simulink model "wlan80211BeaconRx"  (R2018a)
settings: Solver=FixedStepDiscrete  StartTime=0.0  StopTime=Inf  RelTol=1e-3
InitFcn:
  | wlan80211BeaconRxModelParams
  | load('wlan80211BusTypes.mat')
StartFcn:
  | wlan80211BeaconRxModelParams
  | load('wlan80211BusTypes.mat')
model workspace: external: MAT-File (data not in the file)
values from neighbouring files (symbols this model uses):
  p80211 = commwlan80211BeaconRxInit(agcStepSize, agcMaxGain,      corrThreshold, sampsPerChip)    [wlan80211BeaconRxModelParams.m]
libraries: commwlan80211BeaconLib x3, commsync2 x2, commdigbbndpm3 x1, commsequence2 x1, commrfcorlib x1, dspsigops x1, commfilt2 x1
CloseFcn:
  | hFig = findall(0, 'Type', 'figure', 'Name', '802.11 Beacon Frame');
  | if ishghandle(hFig)
  | close(hFig);
  | end
  | clear hFig
  | if (exist('ans')==1) && (iscell(ans) && (numel(ans) == 0))
  | clear ans
  | end
Description:
  | IEEE 802.11 WLAN Beacon Frame Receiver for Captured Data
  | 
  | This example shows how to process a captured beacon frame and display the
  | frame information.
settings Model: Creator=The MathWorks, Inc.  LastModifiedBy=minh
settings DataIOCC: LimitDataPoints=on  SaveFormat=Array  SaveOutput=off  SignalLogging=off  DSMLogging=off  SaveTime=off
settings OptimizationCC: DefaultParameterBehavior=Inlined  InlineInvariantSignals=on  ExpressionDepthLimit=2147483647  EfficientFloat2IntCast=on  LifeSpan=inf
settings DebuggingCC: UnderspecifiedInitializationDetection=Classic  MergeDetectMultiDrivingBlocksExec=none  SolverPrmCheckMsg=warning  UniqueDataStoreMsg=error  AllowSymbolicDim=off  StateNameClashWarn=warning  SFUnexpectedBacktrackingDiag=warning  SFNoUnconditionalDefaultTransitionDiag=warning  SFExecutionAtInitializationDiag=none
settings HardwareCC: ProdBitPerPointer=32  ProdBitPerSizeT=32  ProdBitPerPtrDiffT=32  ProdLargestAtomicFloat=None  ProdIntDivRoundTo=Undefined  ProdEndianess=Unspecified  ProdWordSize=32  ProdHWDeviceType=32-bit Generic
settings ModelReferenceCC: PropagateSignalLabelsOutOfModel=off
settings CodeAppCC: StateflowObjectComments=on
settings GRTTargetCC: TargetLangStandard=C89/C90 (ANSI)  GeneratePreprocessorConditionals=Disable all  CombineOutputUpdateFcns=off  GRTInterface=on
settings ConfigComp: CovMetricSettings=dw  CovHtmlReporting=on  CovSaveCumulativeToWorkspaceVar=on  CovSaveSingleToWorkspaceVar=on  CovShowResultsExplorer=off  CovExternalEMLEnable=off  CovSFcnEnable=off

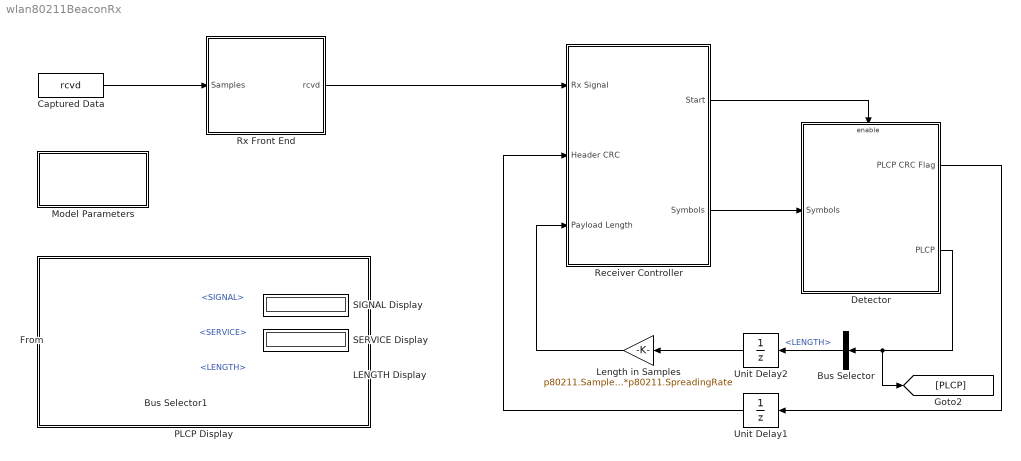
== system wlan80211BeaconRx ==
  Bus Selector : BusSelector  OutputSignals=LENGTH
  Bus Selector1 : BusSelector  OutputSignals=SIGNAL,SERVICE,LENGTH
  Captured Data : FromWorkspace  VariableName=rcvd  SampleTime=p80211.SamplesPerChannelFrame / (p80211.ChipRate*p80211.SamplesPerChip)  Interpolate=off  OutputAfterFinalValue=Cyclic repetition
  Detector : Subsystem
      settings: CloseFcn=clear BeaconFrameBodyType rcvd
  LENGTH Display : Display
  Length in Samples : Gain  Gain=p80211.SamplesPerChip*p80211.SpreadingRate  OutDataTypeStr=uint32  SaturateOnIntegerOverflow=on  ParamDataTypeStr=Inherit: Same as input
  Model Parameters : Subsystem  mask(Model Parameters){rcvdSignal=Channel 5, agcStepSize=6, agcMaxGain=60, corrThreshold=500, sampsPerChip=2}
      mask prompts: rcvdSignal "Received signal:"; agcStepSize "AGC loop gain:"; agcMaxGain "Maximum AGC power gain in dB:"; corrThreshold "Synchronization threshold:"; sampsPerChip "Samples per chip:"
      mask help:
      | Choose 802.11 receiver parameters.
      |
      | You can select from four different saved received signals that contain 802.11 packets captured using a radio.
      |
      | You can set the AGC parameters and samples per chip used in the receiver. You can also set the synchronization threshold value to determine the correlation threshold used to declare the presence of an 802.11 packet.
      mask init:
      | commwlan80211BeaconRxModelParams('init');
      mask Help: helpview(commdhelp);
      mask TypeOptions rcvdSignal: Channel 5 | Channel 9
      mask TypeOptions sampsPerChip: 4 | 2
      mask Display: disp('Model\nParameters')
  PLCP Display : Subsystem
      mask Display: disp('')
  Receiver Controller : Subsystem
  Rx Front End : Subsystem
  SERVICE Display : Display
      settings: Format=hex (Stored Integer)
  SIGNAL Display : Display
      settings: Format=hex (Stored Integer)
  Unit Delay1 : UnitDelay  InitialCondition=1  SampleTime=-1
  Unit Delay2 : UnitDelay  InitialCondition=1  SampleTime=-1
  wires:
  Length in Samples/1 -> Receiver Controller/3(Payload Length)
  Detector/1(PLCP CRC Flag) -> Unit Delay1/1
  Unit Delay1/1 -> Receiver Controller/2(Header CRC)
  Bus Selector/1 -> Unit Delay2/1  "<LENGTH>"
  Receiver Controller/1(Start) -> Detector/Enable
  Rx Front End/1(rcvd) -> Receiver Controller/1(Rx Signal)
  Unit Delay2/1 -> Length in Samples/1
  Detector/2(PLCP) -> [PLCP], Bus Selector/1
  [PLCP] -> Bus Selector1/1
  Bus Selector1/3 -> LENGTH Display/1  "<LENGTH>"
  Bus Selector1/1 -> SIGNAL Display/1  "<SIGNAL>"
  Bus Selector1/2 -> SERVICE Display/1  "<SERVICE>"
  Receiver Controller/2(Symbols) -> Detector/1(Symbols)
  Captured Data/1 -> Rx Front End/1(Samples)

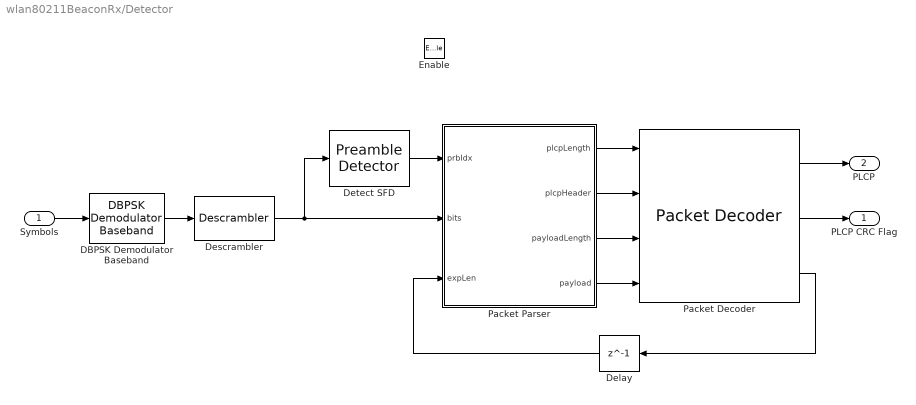
== system wlan80211BeaconRx/Detector ==
  Symbols : Inport
  Enable : EnablePort  StatesWhenEnabling=reset  PropagateVarSize=During execution
  DBPSK Demodulator Baseband : commdigbbndpm3/DBPSK Demodulator Baseband  Ph=0  outDtype=Smallest unsigned integer
      settings: SourceProductName=Communications System Toolbox  SourceProductBaseCode=CM
  Delay : Delay  DelayLength=1  InitialCondition=0  InputProcessing=Columns as channels (frame based)
  Descrambler : commsequence2/Descrambler  M=2  poly=p80211.ScramblerPolynomial  iniStaSource=Dialog Parameter  ini_sta=[0 0 0 0 0 0 0]  resetViaPort=off
      settings: SourceProductName=Communications System Toolbox  SourceProductBaseCode=CM
  Detect SFD : commsync2/Preamble Detector  Input=Bit  Preamble=p80211.SFD  Threshold=3  DetectionMetricOutput=off  Detections=All  SimulateUsing=Code generation
      settings: SourceProductName=Communications System Toolbox  SourceProductBaseCode=CM
  Packet Decoder : commwlan80211BeaconLib/Packet Decoder
      settings: SourceProductName=Communications System Toolbox  SourceProductBaseCode=CM
  Packet Parser : MATLAB Function  TreatAsAtomicUnit=on
  PLCP CRC Flag : Outport  InitialOutput=1
  PLCP : Outport  Port=2
  wires:
  Packet Decoder/3 -> Delay/1
  Packet Decoder/2 -> PLCP CRC Flag/1
  Packet Decoder/1 -> PLCP/1
  Packet Parser/4(payload) -> Packet Decoder/4
  Packet Parser/3(payloadLength) -> Packet Decoder/3
  Packet Parser/2(plcpHeader) -> Packet Decoder/2
  Packet Parser/1(plcpLength) -> Packet Decoder/1
  Delay/1 -> Packet Parser/3(expLen)
  Symbols/1 -> DBPSK Demodulator Baseband/1
  DBPSK Demodulator Baseband/1 -> Descrambler/1
  Detect SFD/1 -> Packet Parser/1(prbIdx)
  Descrambler/1 -> Detect SFD/1, Packet Parser/2(bits)

== system wlan80211BeaconRx/Model Parameters ==

== system wlan80211BeaconRx/PLCP Display ==

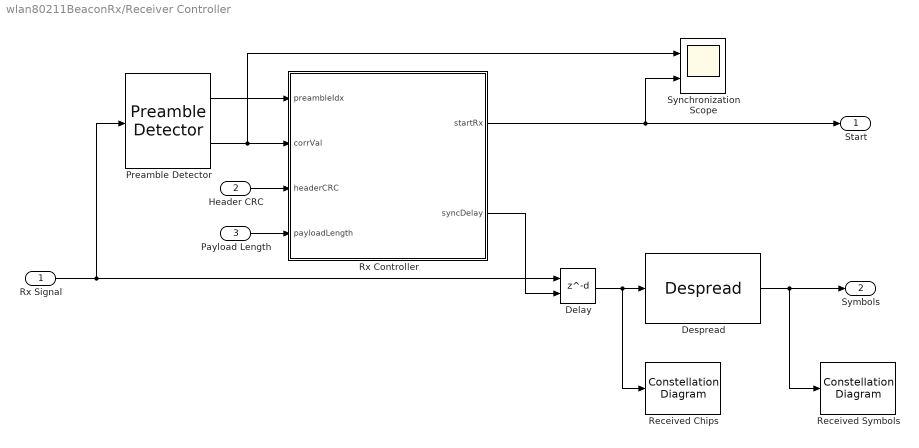
== system wlan80211BeaconRx/Receiver Controller ==
  Rx Signal : Inport
  Header CRC : Inport  Port=2
  Payload Length : Inport  Port=3
  Delay : Delay  DelayLengthSource=Input port  DelayLengthUpperLimit=p80211.SamplesPerChannelFrame  InputProcessing=Columns as channels (frame based)
      settings: InputPortMap=u0,p1
  Despread : commwlan80211BeaconLib/Despread
      settings: SourceProductName=Communications System Toolbox  SourceProductBaseCode=CM
  Preamble Detector : commsync2/Preamble Detector  Input=Symbol  Preamble=p80211.SynchronizationSignal  Threshold=p80211.CorrelationThreshold  DetectionMetricOutput=on  Detections=All  SimulateUsing=Interpreted execution
      settings: SourceProductName=Communications System Toolbox  SourceProductBaseCode=CM
  Received Chips : ConstellationDiagram  Tag=ScatterPlot  Priority=1
  Received Symbols : ConstellationDiagram  Tag=ScatterPlot  Priority=2
  Rx Controller : MATLAB Function  TreatAsAtomicUnit=on
  Synchronization Scope : Scope  NumInputPorts=2
      settings: Priority=1
  Start : Outport
  Symbols : Outport  Port=2
  wires:
  Despread/1 -> Received Symbols/1, Symbols/1
  Rx Controller/2(syncDelay) -> Delay/2
  Rx Controller/1(startRx) -> Synchronization Scope/2, Start/1
  Header CRC/1 -> Rx Controller/3(headerCRC)
  Rx Signal/1 -> Preamble Detector/1, Delay/1
  Payload Length/1 -> Rx Controller/4(payloadLength)
  Delay/1 -> Despread/1, Received Chips/1
  Preamble Detector/2 -> Synchronization Scope/1, Rx Controller/2(corrVal)
  Preamble Detector/1 -> Rx Controller/1(preambleIdx)

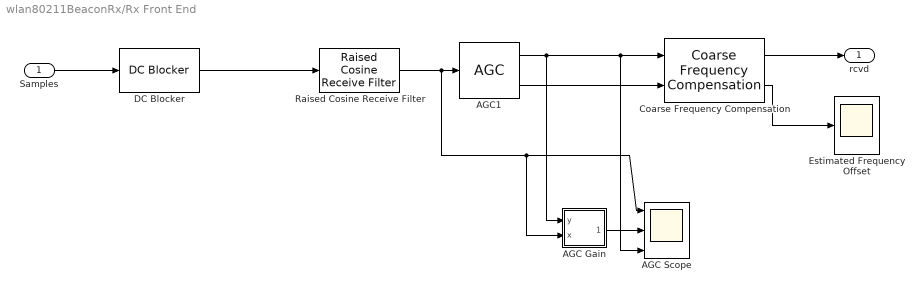
== system wlan80211BeaconRx/Rx Front End ==
  Samples : Inport
  AGC Gain : Subsystem
  AGC Scope : Scope  NumInputPorts=3
  AGC1 : commrfcorlib/AGC  LegacyMode=off  DetectorMethod=Rectifier  LoopMethod=Linear  UpdatePeriod=100  StepSize=0.1  AdaptationStepSize=p80211.AGCStepSize  DesiredOutputPower=1  AveragingLength=50  MaximumGain=30  MaxPowerGain=p80211.AGCUpperLimit  GainOutputPort=off  InputPowerOutputPort=on  SimulateUsing=Code generation
      settings: SourceProductName=Communications System Toolbox
  Coarse Frequency Compensation : commwlan80211BeaconLib/Coarse Frequency Compensation  decimRate=44*p80211.SamplesPerChip/2  maxOffset=50000  M=2
      settings: SourceProductName=Communications System Toolbox  SourceProductBaseCode=CM
  DC Blocker : dspsigops/DC Blocker  Algorithm=IIR  NormalizedBandwidth=0.001  Length=8  Order=6  SimulateUsing=Code generation
      settings: SourceProductName=DSP System Toolbox  SourceProductBaseCode=DS
  Estimated Frequency Offset : Scope
  Raised Cosine Receive Filter : commfilt2/Raised Cosine Receive Filter  filtType=Square root  R=0.3  filtSpan=p80211.FilterOrder  N=p80211.SamplesPerChip  downFactor=1  downOffset=0  filterGain=1  InputProcessing=Columns as channels (frame based)  RateOptions=Enforce single-rate processing  framing=Mute  checkCoeff=off  variableName=rcRxFilt  currentFiltSpan=2*(p80211.FilterOrder/2)  D=p80211.FilterOrder/2  inputOffset=0  sampMode=Mute  saveAsFlag=0  rateMode=Downsampling  checkGain=Normalized  launchFVT=off  roundingMode=Floor  overflowMode=off  coeffDataTypeStr=Inherit: Same word length as input  coeffMin=[]  coeffMax=[]  coeffLastDataTypeStr=Inherit: Same word length as input  accumDataTypeStr=Inherit: Same as product output  accumLastDataTypeStr=Inherit: Same as product output  outputDataTypeStr=Inherit: Same as accumulator  outputMin=[]  outputMax=[]  outputLastDataTypeStr=Inherit: Same as accumulator
  rcvd : Outport
  wires:
  Coarse Frequency Compensation/1 -> rcvd/1
  Samples/1 -> DC Blocker/1
  Raised Cosine Receive Filter/1 -> AGC1/1, AGC Gain/2(x), AGC Scope/1
  AGC1/1 -> AGC Gain/1(y), AGC Scope/3, Coarse Frequency Compensation/1
  AGC Gain/1(gain) -> AGC Scope/2
  Coarse Frequency Compensation/2 -> Estimated Frequency Offset/1
  AGC1/2 -> Coarse Frequency Compensation/2
  DC Blocker/1 -> Raised Cosine Receive Filter/1

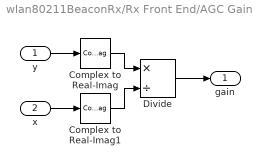
== system wlan80211BeaconRx/Rx Front End/AGC Gain ==
  y : Inport
  x : Inport  Port=2
  Complex to Real-Imag : ComplexToRealImag  Output=Real
  Complex to Real-Imag1 : ComplexToRealImag  Output=Real
  Divide : Product  Inputs=*/
  gain : Outport
  wires:
  Complex to Real-Imag/1 -> Divide/1
  x/1 -> Complex to Real-Imag1/1
  y/1 -> Complex to Real-Imag/1
  Complex to Real-Imag1/1 -> Divide/2
  Divide/1 -> gain/1

== matlab function wlan80211BeaconRx/Detector/Packet Parser ==
  data: prbIdx input; plcpLength output; plcpHeader output size=[p80211.PLCPHeaderLength 1]; payloadLength output; bits input; expLen input; p80211 parameter; payload output size=[p80211.PayloadBufferLength 1]
function [plcpLength, plcpHeader, payloadLength, payload] = ...
  parsePacket(prbIdx, bits, expLen, p80211)

%#codegen

persistent plcpCount payloadCount plcpBuffer payloadBuffer controllerState

% State enums
SearchSFD      = 0;
ReceivePLCP    = 1;
ReceivePayload = 2;


if isempty(plcpCount)
  plcpCount = uint16(1);
  payloadCount = uint16(1);
  % 8 extra bits for synchronizing descrambler
  plcpBuffer = false(p80211.PLCPHeaderLength, 1);
  payloadBuffer = false(p80211.PayloadBufferLength, 1);
  controllerState = SearchSFD;
end

inputLen = uint16(length(bits));
plcpBufferLen = uint16(length(plcpBuffer));
payloadLength = uint16(1);

switch controllerState
  case SearchSFD
    if ~isempty(prbIdx)
      preambleIdx = prbIdx(1);  
      numPLCPBits = inputLen-preambleIdx-1;
      if numPLCPBits >= plcpBufferLen
        plcpBuffer(:) = bits(preambleIdx+(1:plcpBufferLen));
        plcpCount = plcpCount + plcpBufferLen;
        payloadBuffer(1:inputLen-plcpBufferLen-preambleIdx) = ...
          bits(plcpBufferLen+preambleIdx+1:end);
        controllerState = ReceivePayload;
        payloadCount = inputLen-plcpBufferLen-preambleIdx+1;
      else
        plcpBuffer(1:numPLCPBits) = bits(preambleIdx+(1:numPLCPBits));
        plcpCount = plcpCount + numPLCPBits;
        controllerState = ReceivePLCP;
      end
    end
  case ReceivePLCP
    plcpLen = p80211.PLCPHeaderLength;
    if (plcpCount + inputLen) < plcpLen
      plcpBuffer(plcpCount + (1:inputLen)) = bits;
      plcpCount = plcpCount + inputLen;
    else
      plcpBuffer(plcpCount:end) = bits(1:plcpLen-plcpCount+1);
      payloadBuffer(1:inputLen-(plcpLen-plcpCount+1)) = ...
        bits(plcpLen-plcpCount+2:end);
      controllerState = ReceivePayload;
    end
  case ReceivePayload
    payloadBuffer(payloadCount+(0:inputLen-1)) = bits;
    payloadCount = payloadCount + inputLen;
    payloadLength = payloadCount - 1;
    if payloadCount > expLen
      controllerState = SearchSFD;
      plcpCount = uint16(1);
      payloadCount = uint16(1);
    end
end

plcpLength = plcpCount - 1;
plcpHeader = plcpBuffer;
payload = payloadBuffer;

== matlab function wlan80211BeaconRx/Receiver Controller/Rx Controller ==
  data: preambleIdx input; corrVal input; startRx output; headerCRC input boolean size=[1 1]; payloadLength input size=1; p80211 parameter; syncDelay output
function [startRx, syncDelay] = ...
  rxCtrl(preambleIdx, corrVal, headerCRC, payloadLength, p80211)
%#codegen

persistent rxOn controllerState payloadCount lastSyncDelay corrPeakValOld

% State Enums
SearchPLCP = 0;
GetPLCP    = 2;
GetPayload = 4;

if isempty(rxOn)
  % Initialize receiver controller
  rxOn = false;
  controllerState = SearchPLCP;
  payloadCount = 0;
  lastSyncDelay = 0;
  corrPeakValOld = 0;
end

if isempty(preambleIdx)
    corrPeakVal = 0;
    preambleDetected = false;
else
    corrPeakVal = corrVal(preambleIdx(1));
    preambleDetected = true;
end

if (corrPeakValOld < corrPeakVal)
  controllerState = SearchPLCP;
end

switch controllerState
  case SearchPLCP
    % Search for the PLCP SYNC signal
    
    if preambleDetected
      corrPeakValOld = corrPeakVal;
      % Synchronize to the end of the SYNC. Get 8 (scrambler length) extra
      % bits to initialize DPSK demodulator and scrambler
      scramblerLen = length(p80211.ScramblerPolynomial);
      lastSyncDelay = p80211.SamplesPerChannelFrame - (preambleIdx(1) ...
        - scramblerLen*p80211.SpreadingRate*p80211.SamplesPerChip); 
      payloadCount = p80211.NumSYNCSamples ...
        - scramblerLen*p80211.SpreadingRate*p80211.SamplesPerChip;
      rxOn = true;
      
      controllerState = GetPLCP;
    end
  case GetPLCP
    % In this state we receive both SFD, which is part of PLCP preamble,
    % and the PLCP header
    
    payloadCount = payloadCount + p80211.SamplesPerChannelFrame;
    
    if (payloadCount >= ...
        (p80211.NumPLCPSamples+p80211.ScramblerAmbiguitySamples))
    % Wait one more channel frame to let the PLCP CRC result to reach.
    % There is a delay between detector and receiver controller to break
    % the algebraic loop.
      if headerCRC ~= 1
        controllerState = GetPayload;
      else
        rxOn = false;
        lastSyncDelay = 0;
        payloadCount = 0;
        controllerState = SearchPLCP;
      end
    end
  case GetPayload
    % Receive payload symbols
    
    payloadCount = payloadCount + p80211.SamplesPerChannelFrame;
    
    if payloadCount >= ...
        ((p80211.NumPLCPSamples+p80211.ScramblerAmbiguitySamples) + ...
        payloadLength)
      rxOn = false;
      lastSyncDelay = 0;
      payloadCount = 0;
      controllerState = SearchPLCP;
    end
end

startRx = rxOn;
syncDelay = lastSyncDelay;
